simulink model "MPC_X2Constraints"  (Simulink 10.3)
settings: Solver=FixedStepDiscrete  StartTime=0.0  StopTime=tsim  FixedStep=Ts  RelTol=1e-3  EnableMultiTasking=on
values from neighbouring files (symbols this model uses):
  C_states = eye(4)    [Razzo27.m]
  D_states = [0; 0; 0; 0]    [Razzo27.m]
  N = SetN(3)    [Razzo27.m]
  P_MPC = P_d    [Razzo27.m]
  Q_MPC = Q_d    [Razzo27.m]
  R_MPC = R_d    (= 100)    [Razzo27.m]
  sat_max = deg2rad(15)    [Razzo27.m]
  sat_min = deg2rad(-15)    [Razzo27.m]
  sysd = c2d(sys,Ts)    [Razzo27.m]
  Ts = 0.5*(T_taglio/2)    [Razzo27.m]
  x0 = [deg2rad(0) deg2rad(-15) 0 200]    [Razzo27.m]
  x2_max = deg2rad(20)    [Razzo27.m]
  x2_min = deg2rad(-20)    [Razzo27.m]
  x_ref = [0 0 0 0]'    [Razzo27.m]
undefined symbols (not defined in the file or in its folder): MPCInputConstraints, MPCwithX2Constraints
settings Model: Creator=Mirko  LastModifiedBy=dadel  MultithreadedSim=on
settings DataIOCC: LimitDataPoints=on
settings GRTTargetCC: CombineOutputUpdateFcns=on  GRTInterface=off
settings ConfigComp: CovSFcnEnable=off

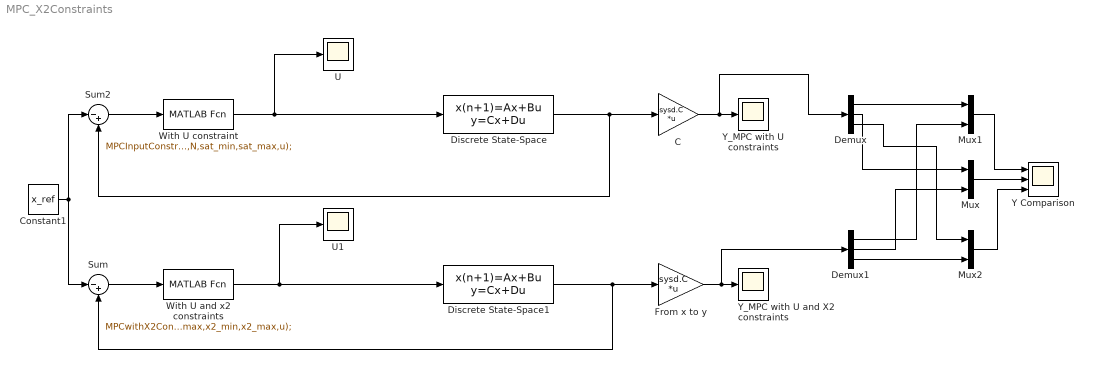
== system MPC_X2Constraints ==
  C : Gain  Gain=sysd.C  Multiplication=Matrix(K*u)
  Constant1 : Constant  Value=x_ref
  Demux : Demux  Outputs=3
  Demux1 : Demux  Outputs=3
  Discrete State-Space : DiscreteStateSpace  A=sysd.A  B=sysd.B  C=C_states  D=D_states  InitialCondition=x0  SampleTime=Ts
  Discrete State-Space1 : DiscreteStateSpace  A=sysd.A  B=sysd.B  C=C_states  D=D_states  InitialCondition=x0  SampleTime=Ts
  From x to y : Gain  Gain=sysd.C  Multiplication=Matrix(K*u)
  Mux : Mux  Inputs=2
  Mux1 : Mux  Inputs=2
  Mux2 : Mux  Inputs=2
  Sum : Sum  Inputs=|-+
  Sum2 : Sum  Inputs=|-+
  U : Scope
  U1 : Scope
  With U and x2 constraints : MATLABFcn  MATLABFcn=MPCwithX2Constraints(sysd.A,sysd.B,Q_MPC,R_MPC,P_MPC,N,sat_min,sat_max,x2_min,x2_max,u);  OutputDimensions=1
  With U constraint : MATLABFcn  MATLABFcn=MPCInputConstraints(sysd.A,sysd.B,Q_MPC,R_MPC,P_MPC,N,sat_min,sat_max,u);  OutputDimensions=1
  Y Comparison : Scope  NumInputPorts=3
  Y_MPC with U and X2 constraints : Scope
  Y_MPC with U constraints : Scope
  wires:
  Discrete State-Space1/1 -> Sum/2, From x to y/1
  Sum/1 -> With U and x2 constraints/1
  From x to y/1 -> Y_MPC with U and X2 constraints/1, Demux1/1
  With U and x2 constraints/1 -> Discrete State-Space1/1, U1/1
  With U constraint/1 -> Discrete State-Space/1, U/1
  Sum2/1 -> With U constraint/1
  Discrete State-Space/1 -> C/1, Sum2/2
  Demux/1 -> Mux1/1
  Mux1/1 -> Y Comparison/1
  Demux1/1 -> Mux1/2
  Demux/2 -> Mux/1
  Demux1/2 -> Mux/2
  Demux1/3 -> Mux2/2
  Demux/3 -> Mux2/1
  Mux2/1 -> Y Comparison/3
  Mux/1 -> Y Comparison/2
  C/1 -> Y_MPC with U constraints/1, Demux/1
  Constant1/1 -> Sum/1, Sum2/1
